simulink model "Controller"  (R2017a)
settings: Solver=VariableStepAuto  StartTime=0.0  StopTime=10.0  RelTol=1e-3
values from neighbouring files (symbols this model uses):
  k1 = a    (= 1)    [evalOriginSensordata.m]
  k2 = a    (= 1)    [evalOriginSensordata.m]
  k3 = a    (= 1)    [evalOriginSensordata.m]
  k4 = a    (= 1)    [evalOriginSensordata.m]
  k5 = a    (= 1)    [evalOriginSensordata.m]
  k6 = a    (= 1)    [evalOriginSensordata.m]
  k7 = a    (= 1)    [evalOriginSensordata.m]
  k8 = a    (= 1)    [evalOriginSensordata.m]
  Ts = 0.05    [startControllerNL.m]
undefined symbols (not defined in the file or in its folder): x
libraries: simulink x3, dspinverses x1, sharedTrackingLibrary x1
settings Model: Creator=Schalker  LastModifiedBy=Schalker

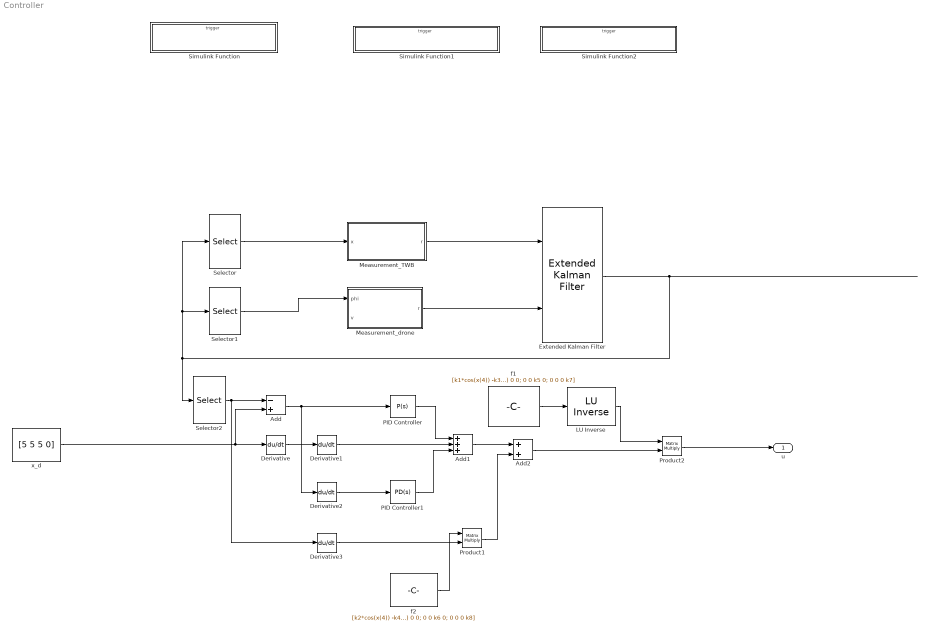
== system Controller ==
  " LU Inverse" : dspinverses/ LU Inverse
      settings: SourceProductName=DSP System Toolbox
  Add : Sum  Inputs=-+
  Add1 : Sum  Inputs=+++
  Add2 : Sum
  Derivative{,1..3} (4 alike) : Derivative
  Extended Kalman Filter : sharedTrackingLibrary/Extended Kalman Filter  StateTransitionFcn=stateTransitionFcn  HasStateTransitionJacobianFcn=off  HasAdditiveProcessNoise=Nonadditive  ProcessNoise=1  HasTimeVaryingProcessNoise=off  HasStateTransitionFcnExtraArgument=0  InitialState=0  InitialStateCovariance=1  MeasurementFcn1=measurementTWBFcn  HasMeasurementJacobianFcn1=off  HasMeasurementEnablePort1=off  HasAdditiveMeasurementNoise1=Nonadditive  MeasurementNoise1=1  HasTimeVaryingMeasurementNoise1=off  HasMeasurementFcnExtraArgument1=0  MeasurementFcn2=measurementDroneFcn  HasMeasurementJacobianFcn2=off  HasMeasurementEnablePort2=off  HasAdditiveMeasurementNoise2=Nonadditive  MeasurementNoise2=1  HasTimeVaryingMeasurementNoise2=off  HasMeasurementFcnExtraArgument2=0  MeasurementFcn3=myMeasurementFcn  HasMeasurementJacobianFcn3=off  HasMeasurementEnablePort3=off  HasAdditiveMeasurementNoise3=Additive  MeasurementNoise3=1  HasTimeVaryingMeasurementNoise3=off  HasMeasurementFcnExtraArgument3=0  MeasurementFcn4=myMeasurementFcn  HasMeasurementJacobianFcn4=off  HasMeasurementEnablePort4=off  HasAdditiveMeasurementNoise4=Additive  MeasurementNoise4=1  HasTimeVaryingMeasurementNoise4=off  HasMeasurementFcnExtraArgument4=0  MeasurementFcn5=myMeasurementFcn  HasMeasurementJacobianFcn5=off  HasMeasurementEnablePort5=off  HasAdditiveMeasurementNoise5=Additive  MeasurementNoise5=1  HasTimeVaryingMeasurementNoise5=off  HasMeasurementFcnExtraArgument5=0  EnableMultirate=on  StateTransitionFcnSampleTime=8  MeasurementFcn1SampleTime=6  MeasurementFcn2SampleTime=1  MeasurementFcn3SampleTime=1  MeasurementFcn4SampleTime=1  MeasurementFcn5SampleTime=1  UseCurrentEstimator=on  OutputStateCovariance=off  DataType=double  SampleTime=1  NumberOfMeasurements=2
  Measurement_TWB : Subsystem
  "Measurement_drone " : Subsystem
  PID Controller : simulink/Continuous/PID Controller  Controller=P  TimeDomain=Continuous-time  SampleTime=-1  IntegratorMethod=Forward Euler  FilterMethod=Forward Euler  Form=Parallel  UseFilter=on  ControllerParametersSource=internal  P=1  I=1  D=0  N=100  InitialConditionSource=internal  InitialConditionForIntegrator=0  InitialConditionForFilter=0  ExternalReset=none  LimitOutput=off  UpperSaturationLimit=inf  LowerSaturationLimit=-inf  LinearizeAsGain=on  AntiWindupMode=none  Kb=1  TrackingMode=off  Kt=1  PParamMin=[]  PParamMax=[]  IParamMin=[]  IParamMax=[]  DParamMin=[]  DParamMax=[]  NParamMin=[]  NParamMax=[]  KbParamMin=[]  KbParamMax=[]  KtParamMin=[]  KtParamMax=[]  POutMin=[]  POutMax=[]  IOutMin=[]  IOutMax=[]  DOutMin=[]  DOutMax=[]  NOutMin=[]  NOutMax=[]  KbOutMin=[]  KbOutMax=[]  KtOutMin=[]  KtOutMax=[]  IntegratorOutMin=[]  IntegratorOutMax=[]  FilterOutMin=[]  FilterOutMax=[]  SumOutMin=[]  SumOutMax=[]  SumI1OutMin=[]  SumI1OutMax=[]  SumI2OutMin=[]  SumI2OutMax=[]  SumI3OutMin=[]  SumI3OutMax=[]  SumDOutMin=[]  SumDOutMax=[]  SaturationOutMin=[]  SaturationOutMax=[]  IntegratorContinuousStateAttributes=''  IntegratorStateMustResolveToSignalObject=off  IntegratorRTWStateStorageClass=Auto  FilterContinuousStateAttributes=''  FilterStateMustResolveToSignalObject=off  FilterRTWStateStorageClass=Auto  DifferentiatorICPrevScaledInput=0  DifferentiatorOutMin=[]  DifferentiatorOutMax=[]  InitialConditionSetting=State (most efficient)
  PID Controller1 : simulink/Continuous/PID Controller  Controller=PD  TimeDomain=Continuous-time  SampleTime=-1  IntegratorMethod=Forward Euler  FilterMethod=Forward Euler  Form=Parallel  UseFilter=on  ControllerParametersSource=internal  P=1  I=1  D=0  N=100  InitialConditionSource=internal  InitialConditionForIntegrator=0  InitialConditionForFilter=0  ExternalReset=none  LimitOutput=off  UpperSaturationLimit=inf  LowerSaturationLimit=-inf  LinearizeAsGain=on  AntiWindupMode=none  Kb=1  TrackingMode=off  Kt=1  PParamMin=[]  PParamMax=[]  IParamMin=[]  IParamMax=[]  DParamMin=[]  DParamMax=[]  NParamMin=[]  NParamMax=[]  KbParamMin=[]  KbParamMax=[]  KtParamMin=[]  KtParamMax=[]  POutMin=[]  POutMax=[]  IOutMin=[]  IOutMax=[]  DOutMin=[]  DOutMax=[]  NOutMin=[]  NOutMax=[]  KbOutMin=[]  KbOutMax=[]  KtOutMin=[]  KtOutMax=[]  IntegratorOutMin=[]  IntegratorOutMax=[]  FilterOutMin=[]  FilterOutMax=[]  SumOutMin=[]  SumOutMax=[]  SumI1OutMin=[]  SumI1OutMax=[]  SumI2OutMin=[]  SumI2OutMax=[]  SumI3OutMin=[]  SumI3OutMax=[]  SumDOutMin=[]  SumDOutMax=[]  SaturationOutMin=[]  SaturationOutMax=[]  IntegratorContinuousStateAttributes=''  IntegratorStateMustResolveToSignalObject=off  IntegratorRTWStateStorageClass=Auto  FilterContinuousStateAttributes=''  FilterStateMustResolveToSignalObject=off  FilterRTWStateStorageClass=Auto  DifferentiatorICPrevScaledInput=0  DifferentiatorOutMin=[]  DifferentiatorOutMax=[]  InitialConditionSetting=State (most efficient)
  Product1 : Product  Multiplication=Matrix(*)
  Product2 : Product  Multiplication=Matrix(*)
  Selector : Selector  InputPortWidth=8  IndexOptions=Index vector (dialog)  Indices=[1 2 3]  OutputSizes=1
  Selector1 : Selector  InputPortWidth=8  IndexOptions=Index vector (dialog)  Indices=[4]  OutputSizes=1
  Selector2 : Selector  InputPortWidth=8  IndexOptions=Index vector (dialog)  Indices=[1:4]  OutputSizes=1
  Simulink Function : Subsystem  TreatAsAtomicUnit=on
  Simulink Function1 : Subsystem  TreatAsAtomicUnit=on
  Simulink Function2 : Subsystem  TreatAsAtomicUnit=on
  "f1 " : Constant  Value=[k1*cos(x(4)) -k3*sin(x(4)) 0 0; k1*sin(x(4)) k3*cos(x(4)) 0 0; 0 0 k5 0; 0 0 0 k7]
  f2 : Constant  Value=[k2*cos(x(4)) -k4*sin(x(4)) 0 0; k2*sin(x(4)) k4*cos(x(4)) 0 0; 0 0 k6 0; 0 0 0 k8]
  "x_d " : Constant  Value=[5 5 5 0]
  u : Outport
  wires:
  Measurement_TWB/1(r) -> Extended Kalman Filter/1
  Extended Kalman Filter/1 -> Selector2/1, Selector1/1, Selector/1
  Selector/1 -> Measurement_TWB/1(x)
  "Measurement_drone "/1(r) -> Extended Kalman Filter/2
  Selector1/1 -> "Measurement_drone "/1(phi)
  Derivative/1 -> Derivative1/1
  "x_d "/1 -> Add/2, Derivative/1
  Add/1 -> Derivative2/1, PID Controller/1
  PID Controller1/1 -> Add1/3
  PID Controller/1 -> Add1/1
  Derivative1/1 -> Add1/2
  Derivative2/1 -> PID Controller1/1
  Add1/1 -> Add2/1
  Selector2/1 -> Derivative3/1, Add/1
  " LU Inverse"/1 -> Product2/1
  "f1 "/1 -> " LU Inverse"/1
  Derivative3/1 -> Product1/2
  Product1/1 -> Add2/2
  Add2/1 -> Product2/2
  f2/1 -> Product1/1
  Product2/1 -> u/1

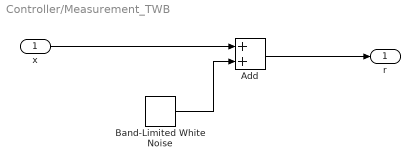
== system Controller/Measurement_TWB ==
  x : Inport
  Add : Sum
  Band-Limited White Noise : simulink/Sources/Band-Limited White Noise  Cov=50  Ts=20*Ts  seed=[23343;23344]
  r : Outport
  wires:
  x/1 -> Add/1
  Add/1 -> r/1
  Band-Limited White Noise/1 -> Add/2

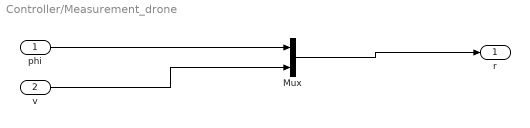
== system Controller/Measurement_drone  ==
  phi : Inport
  v : Inport  Port=2
  Mux : Mux  Inputs=2
  r : Outport
  wires:
  phi/1 -> Mux/1
  Mux/1 -> r/1
  v/1 -> Mux/2

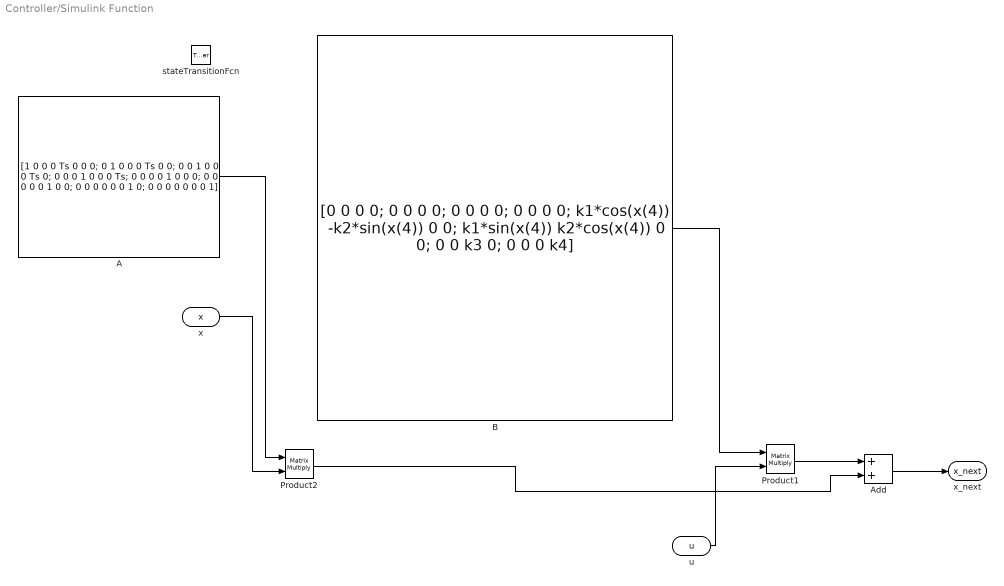
== system Controller/Simulink Function ==
  stateTransitionFcn : TriggerPort  TriggerType=function-call  IsSimulinkFunction=on  FunctionName=stateTransitionFcn  VariantControl=Variant
  A : Constant  Value=|
      | [1 0 0 0 Ts 0 0 0;
      | 0 1 0 0 0 Ts 0 0; 0 0 1 0 0 0 Ts 0;
      | 0 0 0 1 0 0 0 Ts; 0 0 0 0 1 0 0  0; 0 0 0 0 0 1 0 0;
      | 0 0 0 0 0 0 1  0;
      | 0 0 0 0 0 0 0 1]
  Add : Sum
  B : Constant  Value=|
      | [0 0 0 0;
      | 0 0 0 0;
      | 0 0 0 0;
      | 0 0 0 0;
      | k1*cos(x(4)) -k2*sin(x(4)) 0 0;
      | k1*sin(x(4)) k2*cos(x(4)) 0 0;
      | 0 0 k3 0;
      | 0 0 0 k4]
  Product1 : Product  Multiplication=Matrix(*)
  Product2 : Product  Multiplication=Matrix(*)
  x : ArgIn  DisableCoverage=on  ArgumentName=x
  u : ArgIn  DisableCoverage=on  Port=2  PortDimensions=4  ArgumentName=u
  x_next : ArgOut  DisableCoverage=on  PortDimensions=8  ArgumentName=x_next
  wires:
  u/1 -> Product1/2
  x/1 -> Product2/2
  A/1 -> Product2/1
  B/1 -> Product1/1
  Product1/1 -> Add/1
  Add/1 -> x_next/1
  Product2/1 -> Add/2

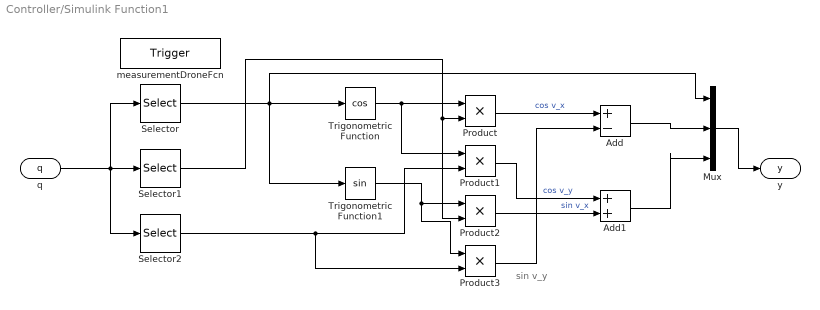
== system Controller/Simulink Function1 ==
  note: sin v_y
  measurementDroneFcn : TriggerPort  TriggerType=function-call  IsSimulinkFunction=on  FunctionName=measurementDroneFcn  VariantControl=Variant
  Add : Sum  Inputs=+-
  Add1 : Sum
  Mux : Mux  Inputs=3
  Product{,1..3} (4 alike) : Product
  Selector : Selector  InputPortWidth=3  IndexOptions=Index vector (dialog)  Indices=[1]  OutputSizes=1
  Selector1 : Selector  InputPortWidth=3  IndexOptions=Index vector (dialog)  Indices=[2]  OutputSizes=1
  Selector2 : Selector  InputPortWidth=3  IndexOptions=Index vector (dialog)  Indices=[3]  OutputSizes=1
  Trigonometric Function : Trigonometry  Operator=cos
  Trigonometric Function1 : Trigonometry
  q : ArgIn  DisableCoverage=on  PortDimensions=3  ArgumentName=q
  y : ArgOut  DisableCoverage=on  PortDimensions=3  ArgumentName=y
  wires:
  q/1 -> Selector2/1, Selector/1, Selector1/1
  Mux/1 -> y/1
  Selector/1 -> Mux/1, Trigonometric Function1/1, Trigonometric Function/1
  Trigonometric Function/1 -> Product1/1, Product/1
  Selector2/1 -> Product1/2, Product3/2
  Trigonometric Function1/1 -> Product3/1, Product2/1
  Selector1/1 -> Product/2, Product2/2
  Product/1 -> Add/1  "cos v_x"
  Add/1 -> Mux/2
  Product1/1 -> Add1/1  "cos v_y"
  Product3/1 -> Add/2
  Product2/1 -> Add1/2  "sin v_x"
  Add1/1 -> Mux/3

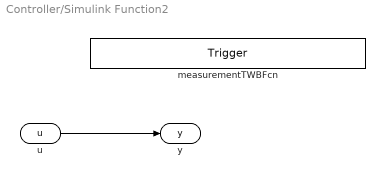
== system Controller/Simulink Function2 ==
  measurementTWBFcn : TriggerPort  TriggerType=function-call  IsSimulinkFunction=on  FunctionName=measurementTWBFcn  VariantControl=Variant
  u : ArgIn  DisableCoverage=on  PortDimensions=3  ArgumentName=u
  y : ArgOut  DisableCoverage=on  PortDimensions=3  ArgumentName=y
  wires:
  u/1 -> y/1
